simulink model "DRPLDM_2015a"  (R2015a)
settings: Solver=ode3  StartTime=0.0  StopTime=TimeVector(end)  FixedStep=Tsim  RelTol=1e-3
values from neighbouring files (symbols this model uses):
  EngUnits = 1    [RunModel.m]
  HILMode = 1    [RunModel.m]
  LeverMode = 1    [RunModel.m]
  Mode = 0    [RunModel.m]
  Mwm = 0.35    [RunModel.m]
  TCFaultSoftSim = 1    [RunModel.m]    (also in SetFaultSim.m)
  WhichCont = 2    [RunModel.m]
  WhichEngine = 1    [RunModel.m]
undefined symbols (not defined in the file or in its folder): FaultStartTime, FaultStopTime
libraries: Lib_Solve_ModelSource_TMATS x5, simulink x3
settings Model: Creator=antoniohadadeneto  LastModifiedBy=anton
settings DataIOCC: LimitDataPoints=off  SaveFormat=Dataset
settings HardwareCC: ProdBitPerPointer=64  ProdLargestAtomicFloat=Float  ProdIntDivRoundTo=Zero  ProdEndianess=LittleEndian  ProdHWDeviceType=Specified
settings GRTTargetCC: GeneratePreprocessorConditionals=Use local settings

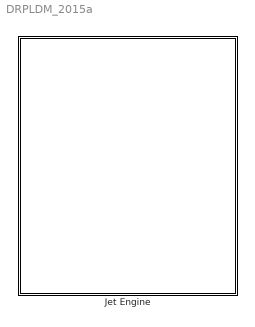
== system DRPLDM_2015a ==
  Jet Engine : Subsystem

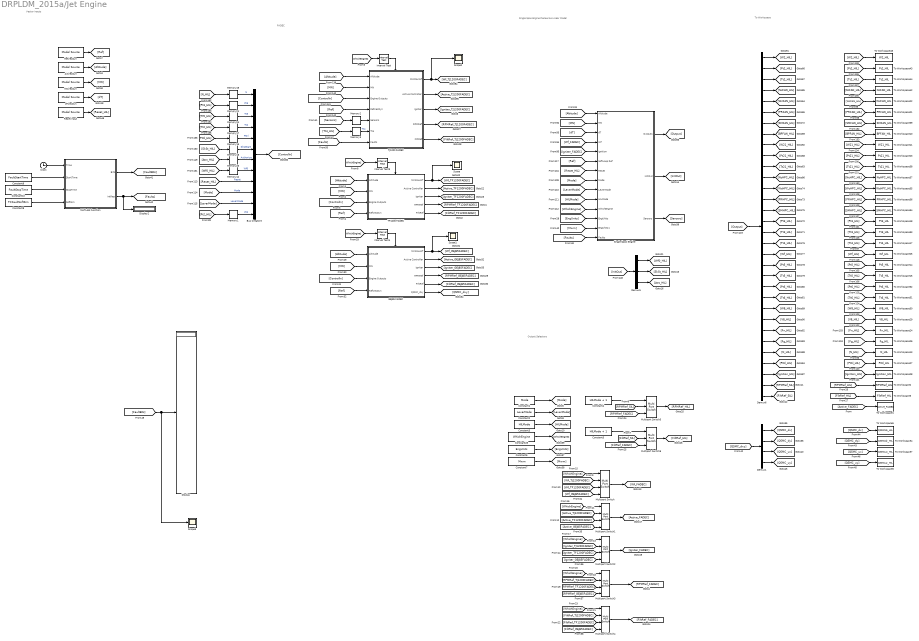
== system DRPLDM_2015a/Jet Engine ==
  note: Vector Inputs
  note: Single Spoo Engine
      | Piecewise
      | Linear Model
  note: To Workspace
  note: Output Selectors
  note: FADEC
  AltVecDyn : Lib_Solve_ModelSource_TMATS/Model Source  T_vec_M=TimeVector  input_array_M=AltVecDyn
  Bus Creator3 : BusCreator  Inputs=12
  Clock : Clock
  Constant1 : Constant  Value=Mode
  Constant10 : Constant  Value=FaultStopTime
  Constant2 : Constant  Value=LeverMode
  Constant25 : Constant  Value=WhichEngine
  Constant3 : Constant  Value=HILMode
  Constant4 : Constant  Value=HILMode + 1
  Constant5 : Constant  Value=HILMode + 1
  Constant6 : Constant  Value=EngUnits
  Constant7 : Constant  Value=Mwm
  Constant8 : Constant  Value=TCFaultSoftSim
  Constant9 : Constant  Value=FaultStartTime
  Demux1 : Demux
  Demux5 : Demux  Outputs=3
  Demux6 : Demux  Outputs=32
  Display : Display
  Display2 : Display
  GEJ85 FADEC : Subsystem  TreatAsAtomicUnit=on
  Interval Test : simulink/Logic and Bit Operations/Interval Test  IntervalClosedRight=on  uplimit=1.5  IntervalClosedLeft=on  lowlimit=0.5  OutDataTypeStr=boolean
  Interval Test3 : simulink/Logic and Bit Operations/Interval Test  IntervalClosedRight=on  uplimit=2.5  IntervalClosedLeft=on  lowlimit=1.5  OutDataTypeStr=boolean
  Interval Test4 : simulink/Logic and Bit Operations/Interval Test  IntervalClosedRight=on  uplimit=3.5  IntervalClosedLeft=on  lowlimit=2.5  OutDataTypeStr=boolean
  MATLAB Function : MATLAB Function  TreatAsAtomicUnit=on
      settings: PermitHierarchicalResolution=ParametersOnly
  MNVecDyn : Lib_Solve_ModelSource_TMATS/Model Source  T_vec_M=TimeVector  input_array_M=MNVecDyn
  Memory{1..3,12,15,17..19,21,24..25} (11 alike) : Memory
  Multiport Switch{,1..4} (5 alike) : MultiPortSwitch
  Multiport Switch5 : MultiPortSwitch  Inputs=2
  Multiport Switch6 : MultiPortSwitch  Inputs=2
  RefVecDyn : Lib_Solve_ModelSource_TMATS/Model Source  T_vec_M=TimeVector  input_array_M=RefVecDyn
  Reset Input : Lib_Solve_ModelSource_TMATS/Model Source  T_vec_M=TimeVector  input_array_M=ResetInput
  Scope{,1..3} (4 alike) : Scope
      Scope settings: TimeRange=auto  MaxDataPoints=5000  SaveToWorkspace=off  YMin=-1.00000  YMax=1.00000  SampleTime=-1
      Scope1 settings: TimeRange=auto  MaxDataPoints=5000  SaveToWorkspace=off  SaveName=ScopeData6  YMin=-0.03827  YMax=0.34443  SampleTime=-1
      Scope2 settings: TimeRange=auto  MaxDataPoints=5000  SaveToWorkspace=off  SaveName=ScopeData7  YMin=-1.00000  YMax=1.00000  SampleTime=-1
      Scope3 settings: TimeRange=auto  MaxDataPoints=5000  SaveToWorkspace=off  YMin=-0.125  YMax=1.125  SampleTime=-1
  Single Spool Engine : Subsystem  TreatAsAtomicUnit=on
  TF1200 FADEC : Subsystem  TreatAsAtomicUnit=on
  TJ1200 FADEC : Subsystem  TreatAsAtomicUnit=on
  To Workspace1 : ToWorkspace  VariableName=Active_FADEC  SampleTime=-1
  To Workspace13 : ToWorkspace  VariableName=N_HIL  SampleTime=-1
  To Workspace14 : ToWorkspace  VariableName=Pt5_HIL  SampleTime=-1
  To Workspace15 : ToWorkspace  VariableName=Tt5_HIL  SampleTime=-1
  To Workspace17 : ToWorkspace  VariableName=Tt4_HIL  SampleTime=-1
  To Workspace18 : ToWorkspace  VariableName=Pt3_HIL  SampleTime=-1
  To Workspace2 : ToWorkspace  VariableName=RPMRef_HIL  SampleTime=-1
  To Workspace21 : ToWorkspace  VariableName=PRFAN_HIL  SampleTime=-1
  To Workspace22 : ToWorkspace  VariableName=WcFAN_HIL  SampleTime=-1
  To Workspace23 : ToWorkspace  VariableName=Pt21_HIL  SampleTime=-1
  To Workspace24 : ToWorkspace  VariableName=Fn_HIL  SampleTime=-1
  To Workspace25 : ToWorkspace  VariableName=Wf_HIL  SampleTime=-1
  To Workspace26 : ToWorkspace  VariableName=Fg_HIL  SampleTime=-1
  To Workspace27 : ToWorkspace  VariableName=POil_HIL  SampleTime=-1
  To Workspace28 : ToWorkspace  VariableName=Ignition_HIL  SampleTime=-1
  To Workspace29 : ToWorkspace  VariableName=V8_HIL  SampleTime=-1
  To Workspace3 : ToWorkspace  VariableName=FiltRef_HIL  SampleTime=-1
  To Workspace30 : ToWorkspace  VariableName=W8_HIL  SampleTime=-1
  To Workspace31 : ToWorkspace  VariableName=Tt6_HIL  SampleTime=-1
  To Workspace32 : ToWorkspace  VariableName=Pt6_HIL  SampleTime=-1
  To Workspace33 : ToWorkspace  VariableName=Tt3_HIL  SampleTime=-1
  To Workspace34 : ToWorkspace  VariableName=SMHPC_HIL  SampleTime=-1
  To Workspace35 : ToWorkspace  VariableName=WcHPC_HIL  SampleTime=-1
  To Workspace36 : ToWorkspace  VariableName=PRHPC_HIL  SampleTime=-1
  To Workspace37 : ToWorkspace  VariableName=NcHPC_HIL  SampleTime=-1
  To Workspace38 : ToWorkspace  VariableName=Tt21_HIL  SampleTime=-1
  To Workspace39 : ToWorkspace  VariableName=SMFAN_HIL  SampleTime=-1
  To Workspace4 : ToWorkspace  VariableName=QSMCdy_HIL  SampleTime=-1
  To Workspace40 : ToWorkspace  VariableName=BPFAN_HIL  SampleTime=-1
  To Workspace41 : ToWorkspace  VariableName=W21_HIL  SampleTime=-1
  To Workspace42 : ToWorkspace  VariableName=NcFAN_HIL  SampleTime=-1
  To Workspace43 : ToWorkspace  VariableName=Pt2_HIL  SampleTime=-1
  To Workspace44 : ToWorkspace  VariableName=Tt2_HIL  SampleTime=-1
  To Workspace45 : ToWorkspace  VariableName=W2_HIL  SampleTime=-1
  To Workspace5 : ToWorkspace  VariableName=QSMCdx_HIL  SampleTime=-1
  To Workspace6 : ToWorkspace  VariableName=QSMCuy_HIL  SampleTime=-1
  To Workspace7 : ToWorkspace  VariableName=QSMCux_HIL  SampleTime=-1
  dTVecDyn : Lib_Solve_ModelSource_TMATS/Model Source  T_vec_M=TimeVector  input_array_M=dTVecDyn
  wires:
  [QSMC_uy] -> To Workspace6/1
  Demux6/29 -> [POil_HIL]
  [Pt5_HIL] -> To Workspace14/1
  Demux6/16 -> [Pt3_HIL]
  [Fn_HIL] -> To Workspace24/1
  [Reset_HIL] -> Single Spool Engine/7(Reset)
  Demux6/15 -> [SMHPC_HIL]
  [WhichEngine] -> Interval Test3/1
  [Wf_HIL] -> To Workspace25/1
  dTVecDyn/1 -> [dT]
  GEJ85 FADEC/2(Active Controller) -> [Active_GEJ85FADEC]
  [Pt3_HIL] -> To Workspace18/1
  Memory19/1 -> Bus Creator3/1  "N"
  [WcFAN_HIL] -> To Workspace22/1
  [NcHPC_HIL] -> To Workspace37/1
  [Tt3_HIL] -> To Workspace33/1
  [Active_FADEC] -> To Workspace1/1
  Interval Test3/1 -> TF1200 FADEC/Enable
  [W21_HIL] -> To Workspace41/1
  [WhichEngine] -> Interval Test/1
  Demux6/30 -> [Ignition_HIL]
  Interval Test/1 -> TJ1200 FADEC/Enable
  [Ignition_HIL] -> To Workspace28/1
  [Pt2_HIL] -> To Workspace43/1
  Constant2/1 -> [LeverMode]
  Memory1/1 -> Bus Creator3/12  "Pt2"
  [MN] -> TJ1200 FADEC/2(MN)
  [QSMC_dxy] -> Demux1/1
  TJ1200 FADEC/3(Igniter) -> [Igniter_TJ1200FADEC]
  [Tt21_HIL] -> To Workspace38/1
  GEJ85 FADEC/4(RPMRef) -> [RPMRef_GEJ85FADEC]
  Demux6/31 -> [RPMRef_SIL]
  Multiport Switch2/1 -> [Igniter_FADEC]
  Demux6/22 -> [Pt6_HIL]
  Constant3/1 -> [HILMode]
  Demux6/21 -> [Tt5_HIL]
  Demux6/17 -> [Tt3_HIL]
  [Pt6_HIL] -> To Workspace32/1
  Demux6/25 -> [V8_HIL]
  [Ref] -> Single Spool Engine/6(SoftLoop Ref)
  [Output] -> Demux6/1
  [N_HIL] -> To Workspace13/1
  Demux6/3 -> [Tt2_HIL]
  Demux6/32 -> [FiltRef_SIL]
  Demux6/23 -> [Tt6_HIL]
  Demux6/13 -> [WcHPC_HIL]
  Memory12/1 -> Bus Creator3/8  "Wf0"
  Multiport Switch/1 -> [Wf_FADEC]
  Memory21/1 -> Bus Creator3/2  "Pt3"
  TJ1200 FADEC/2(Active Controller) -> [Active_TJ1200FADEC]
  Demux6/24 -> [W8_HIL]
  Demux6/19 -> [Wf_HIL]
  [WhichEngine] -> Multiport Switch2/1
  [SMHPC_HIL] -> To Workspace34/1
  [Igniter_TJ1200FADEC] -> Multiport Switch2/2
  Demux6/26 -> [Fn_HIL]
  [Altitude] -> GEJ85 FADEC/1(Altitude)
  [ControlIn] -> TJ1200 FADEC/3(Engine Outputs)
  [Tt6_HIL] -> To Workspace31/1
  [PRHPC_HIL] -> To Workspace36/1
  [NcFAN_HIL] -> To Workspace42/1
  [W2_HIL] -> To Workspace45/1
  [ControlIn] -> TF1200 FADEC/3(Engine Outputs)
  [Tt2_HIL] -> To Workspace44/1
  Interval Test4/1 -> GEJ85 FADEC/Enable
  [FiltRef_TJ1200FADEC] -> Multiport Switch4/2
  [RPMRef_TF1200FADEC] -> Multiport Switch3/3
  Demux5/1 -> [Wf0_HIL]
  [Pt3_HIL] -> Memory21/1
  [Ref] -> TJ1200 FADEC/4(RefVecDyn)
  [ControlIn] -> GEJ85 FADEC/3(Engine Outputs)
  TJ1200 FADEC/1(MinMaxWf) -> Scope2/1, [Wf_TJ1200FADEC]
  [Altitude] -> TJ1200 FADEC/1(Altitude)
  Constant25/1 -> [WhichEngine]
  [LeverMode] -> Bus Creator3/11  "LeverMode"
  Memory25/1 -> Bus Creator3/7  "Authorize"
  [Mode] -> Bus Creator3/10  "Mode"
  [Reset_HIL] -> Bus Creator3/9  "Reset"
  [W8_HIL] -> To Workspace30/1
  [V8_HIL] -> To Workspace29/1
  TF1200 FADEC/1(MinMaxWf) -> Scope/1, [Wf_TF1200FADEC]
  [SMFAN_HIL] -> To Workspace39/1
  Memory15/1 -> Bus Creator3/5  "POil"
  Demux6/28 -> [N_HIL]
  [Wf0_HIL] -> Memory12/1
  TF1200 FADEC/2(Active Controller) -> [Active_TF1200FADEC]
  Demux5/2 -> [SkSt_HIL]
  Demux6/6 -> [PRFAN_HIL]
  [Ref] -> TF1200 FADEC/4(RefVecDyn)
  Memory17/1 -> Bus Creator3/4  "Tt2"
  TF1200 FADEC/3(Igniter) -> [Igniter_TF1200FADEC]
  [N_HIL] -> Memory19/1
  [MN] -> GEJ85 FADEC/2(MN)
  [MN] -> TF1200 FADEC/2(MN)
  Demux6/10 -> [Pt21_HIL]
  GEJ85 FADEC/3(Igniter) -> [Igniter_GEJ85FADEC]
  Demux6/11 -> [Tt21_HIL]
  MNVecDyn/1 -> [MN]
  AltVecDyn/1 -> [Altitude]
  Demux6/12 -> [NcHPC_HIL]
  [RPMRef_TJ1200FADEC] -> Multiport Switch3/2
  [Altitude] -> TF1200 FADEC/1(Altitude)
  Single Spool Engine/1(Outputs) -> [Output]
  [dT] -> Single Spool Engine/3(dT)
  Constant5/1 -> Multiport Switch6/1
  [Tt5_HIL] -> To Workspace15/1
  [Pt21_HIL] -> To Workspace23/1
  [Tt4_HIL] -> To Workspace17/1
  [PRFAN_HIL] -> To Workspace21/1
  [Wf_FADEC] -> Single Spool Engine/4(Wf)
  [Altitude] -> Single Spool Engine/1(Altitude)
  Demux6/1 -> [W2_HIL]
  Demux6/5 -> [WcFAN_HIL]
  [Fg_HIL] -> To Workspace26/1
  Demux6/9 -> [W21_HIL]
  [Mode] -> Single Spool Engine/8(Mode)
  Demux1/3 -> [QSMC_ux]
  [FiltRef_GEJ85FADEC] -> Multiport Switch4/4
  [WhichEngine] -> Interval Test4/1
  [Wf_TF1200FADEC] -> Multiport Switch/3
  TF1200 FADEC/5(FiltRef) -> [FiltRef_TF1200FADEC]
  Constant4/1 -> Multiport Switch5/1
  [WhichEngine] -> Multiport Switch4/1
  [Wf_TJ1200FADEC] -> Multiport Switch/2
  Reset Input/1 -> [Reset_HIL]
  [WhichEngine] -> Multiport Switch3/1
  [WhichEngine] -> Multiport Switch1/1
  [Active_TF1200FADEC] -> Multiport Switch1/3
  [Active_GEJ85FADEC] -> Multiport Switch1/4
  [WhichEngine] -> Multiport Switch/1
  [SkSt_HIL] -> Memory18/1
  [MN] -> Single Spool Engine/2(MN)
  [FiltRef_SIL] -> Multiport Switch6/2
  Memory24/1 -> Bus Creator3/3  "Tt5"
  [RPMRef_SIL] -> Multiport Switch5/2
  Demux5/3 -> [Atrz_HIL]
  [Igniter_FADEC] -> Single Spool Engine/5(Ignition)
  [FiltRef_HIL] -> To Workspace3/1
  [RPMRef_FADEC] -> Multiport Switch5/3
  [WhichEngine] -> Single Spool Engine/11(WhichEngine)
  [Active_TJ1200FADEC] -> Multiport Switch1/2
  [FiltRef_TF1200FADEC] -> Multiport Switch4/3
  [FiltRef_FADEC] -> Multiport Switch6/3
  GEJ85 FADEC/5(FiltRef) -> [FiltRef_GEJ85FADEC]
  TJ1200 FADEC/4(RPMRef) -> [RPMRef_TJ1200FADEC]
  [Igniter_TF1200FADEC] -> Multiport Switch2/3
  TF1200 FADEC/4(RPMRef) -> [RPMRef_TF1200FADEC]
  [POil_HIL] -> To Workspace27/1
  Demux6/7 -> [SMFAN_HIL]
  Demux6/20 -> [Pt5_HIL]
  [WcHPC_HIL] -> To Workspace35/1
  [Ref] -> GEJ85 FADEC/4(RefVecDyn)
  GEJ85 FADEC/1(MinMaxWf) -> Scope1/1, [Wf_GEJ85FADEC]
  Multiport Switch6/1 -> [FiltRef_HIL]
  Multiport Switch3/1 -> [RPMRef_FADEC]
  [Tt5_HIL] -> Memory24/1
  Multiport Switch5/1 -> [RPMRef_HIL]
  [Wf_GEJ85FADEC] -> Multiport Switch/4
  [BPFAN_HIL] -> To Workspace40/1
  Demux6/8 -> [BPFAN_HIL]
  [Atrz_HIL] -> Memory25/1
  Demux6/27 -> [Fg_HIL]
  [Igniter_GEJ85FADEC] -> Multiport Switch2/4
  [RPMRef_GEJ85FADEC] -> Multiport Switch3/4
  [Tt2_HIL] -> Memory17/1
  [QSMC_dy] -> To Workspace4/1
  RefVecDyn/1 -> [Ref]
  Demux1/2 -> [QSMC_dy]
  Demux6/18 -> [Tt4_HIL]
  Demux6/4 -> [NcFAN_HIL]
  Multiport Switch1/1 -> [Active_FADEC]
  Constant1/1 -> [Mode]
  [QSMC_dx] -> To Workspace5/1
  Single Spool Engine/2(InitOut) -> [InitOut]
  Demux6/2 -> [Pt2_HIL]
  [QSMC_ux] -> To Workspace7/1
  GEJ85 FADEC/6(QSMC_dxy) -> [QSMC_dxy]
  Demux1/1 -> [QSMC_dx]
  [InitOut] -> Demux5/1
  Demux1/4 -> [QSMC_uy]
  TJ1200 FADEC/5(FiltRef) -> [FiltRef_TJ1200FADEC]
  Bus Creator3/1 -> [ControlIn]
  Multiport Switch4/1 -> [FiltRef_FADEC]
  [LeverMode] -> Single Spool Engine/9(LeverMode)
  [Pt2_HIL] -> Memory1/1
  Memory18/1 -> Bus Creator3/6  "SkipStart"
  [POil_HIL] -> Memory15/1
  [RPMRef_HIL] -> To Workspace2/1
  Demux6/14 -> [PRHPC_HIL]
  [HILMode] -> Single Spool Engine/10(HILMode)
  Constant6/1 -> [EngUnits]
  [EngUnits] -> Single Spool Engine/12(EngUhits)
  [Mwm] -> Single Spool Engine/13(EngUhits1)
  Constant7/1 -> [Mwm]
  Single Spool Engine/3(Sensors) -> [Sensors]
  [Sensors] -> Memory2/1
  Memory2/1 -> TJ1200 FADEC/5(Sensors)
  Memory3/1 -> TJ1200 FADEC/6(Tt4)  "Tt4"
  [Tt4_HIL] -> Memory3/1
  [Faults] -> Single Spool Engine/14(Faults)
  [FaultBits] -> Scope3/1, Display/1
  Clock/1 -> MATLAB Function/1(Time)
  Constant9/1 -> MATLAB Function/2(StartTime)
  Constant10/1 -> MATLAB Function/3(StopTime)
  MATLAB Function/1(Bits) -> [FaultBits]
  MATLAB Function/2(IntRep) -> [Faults], Display2/1
  [Faults] -> TJ1200 FADEC/7(Faults)
  Constant8/1 -> MATLAB Function/4(SoftSim)

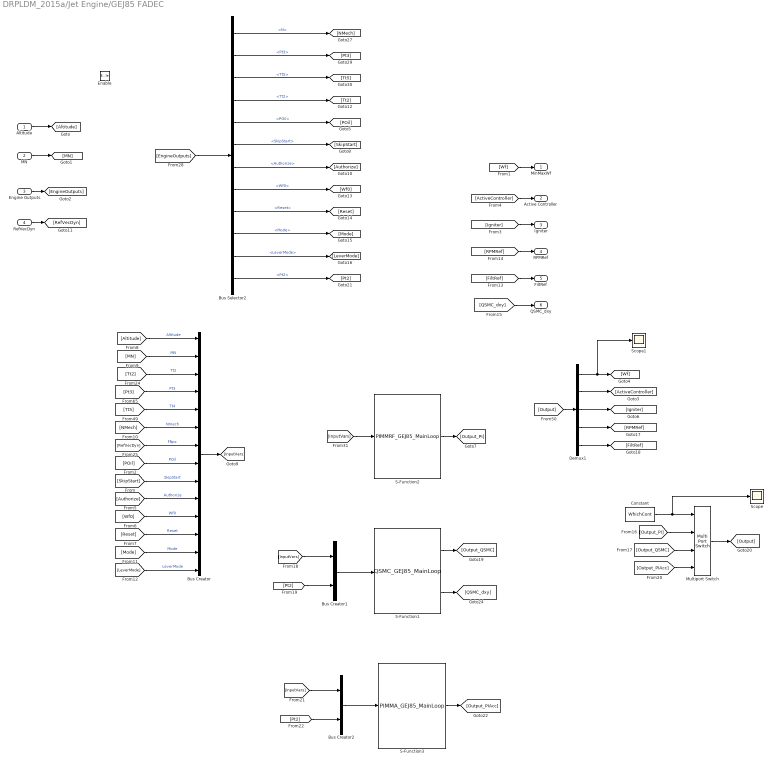
== system DRPLDM_2015a/Jet Engine/GEJ85 FADEC ==
  Altitude : Inport
  MN : Inport  Port=2
  Engine Outputs : Inport  Port=3
  RefVecDyn : Inport  Port=4
  Enable : EnablePort
  Bus Creator : BusCreator  Inputs=14
  Bus Creator1 : BusCreator  Inputs=2
  Bus Creator2 : BusCreator  Inputs=2
  Bus Selector2 : BusSelector  OutputSignals=N,Pt3,Tt5,Tt2,POil,SkipStart,Authorize,Wf0,Reset,Mode,LeverMode,Pt2
  Constant : Constant  Value=WhichCont
  Demux1 : Demux  Outputs=5
  Multiport Switch : MultiPortSwitch
  S-Function1 : S-Function  FunctionName=QSMC_GEJ85_MainLoop  SFunctionDeploymentMode=off  EnableBusSupport=off
  S-Function2 : S-Function  FunctionName=PIMMRF_GEJ85_MainLoop  SFunctionDeploymentMode=off  EnableBusSupport=off
  S-Function3 : S-Function  FunctionName=PIMMA_GEJ85_MainLoop  SFunctionDeploymentMode=off  EnableBusSupport=off
  Scope : Scope
      settings: TimeRange=auto  MaxDataPoints=5000  SaveToWorkspace=off  YMin=1.00000  YMax=3.00000  SampleTime=-1
  Scope1 : Scope
      settings: TimeRange=auto  MaxDataPoints=5000  SaveToWorkspace=off  SaveName=ScopeData2  YMin=-0.03465  YMax=0.31188  SampleTime=-1
  MinMaxWf : Outport
  Active Controller : Outport  Port=2  InitialOutput=0
  Igniter : Outport  Port=3  InitialOutput=0
  RPMRef : Outport  Port=4  InitialOutput=0
  FiltRef : Outport  Port=5  InitialOutput=0
  QSMC_dxy : Outport  Port=6  InitialOutput=0
  wires:
  Demux1/5 -> [FiltRef]
  Demux1/4 -> [RPMRef]
  [FiltRef] -> FiltRef/1
  [RPMRef] -> RPMRef/1
  Bus Selector2/4 -> [Tt2]  "<Tt2>"
  Altitude/1 -> [Altitude]
  MN/1 -> [MN]
  Engine Outputs/1 -> [EngineOutputs]
  RefVecDyn/1 -> [RefVecDyn]
  [EngineOutputs] -> Bus Selector2/1
  Bus Selector2/1 -> [NMech]  "<N>"
  Bus Selector2/2 -> [Pt3]  "<Pt3>"
  Bus Selector2/3 -> [Tt5]  "<Tt5>"
  [Wf] -> MinMaxWf/1
  [ActiveController] -> Active Controller/1
  [Altitude] -> Bus Creator/1  "Altitude"
  [MN] -> Bus Creator/2  "MN"
  Bus Creator/1 -> [InputVars]
  [InputVars] -> S-Function2/1
  S-Function2/1 -> [Output_PI]
  [Output] -> Demux1/1
  Demux1/1 -> Scope1/1, [Wf]
  Demux1/2 -> [ActiveController]
  [Tt2] -> Bus Creator/3  "Tt2"
  [Pt3] -> Bus Creator/4  "Pt3"
  [Tt5] -> Bus Creator/5  "Tt4"
  [NMech] -> Bus Creator/6  "Nmech"
  [RefVecDyn] -> Bus Creator/7  "FNpc"
  Bus Selector2/5 -> [POil]  "<POil>"
  [POil] -> Bus Creator/8  "POil"
  Demux1/3 -> [Igniter]
  [Igniter] -> Igniter/1
  Bus Selector2/6 -> [SkipStart]  "<SkipStart>"
  [SkipStart] -> Bus Creator/9  "SkipStart"
  Bus Selector2/7 -> [Authorize]  "<Authorize>"
  Bus Selector2/8 -> [Wf0]  "<Wf0>"
  [Authorize] -> Bus Creator/10  "Authorize"
  [Wf0] -> Bus Creator/11  "Wf0"
  Bus Selector2/9 -> [Reset]  "<Reset>"
  [Reset] -> Bus Creator/12  "Reset"
  Bus Selector2/10 -> [Mode]  "<Mode>"
  Bus Selector2/11 -> [LeverMode]  "<LeverMode>"
  [Mode] -> Bus Creator/13  "Mode"
  [LeverMode] -> Bus Creator/14  "LeverMode"
  Bus Creator1/1 -> S-Function1/1
  S-Function1/1 -> [Output_QSMC]
  [Output_QSMC] -> Multiport Switch/3
  [Output_PI] -> Multiport Switch/2
  Constant/1 -> Scope/1, Multiport Switch/1
  Multiport Switch/1 -> [Output]
  [InputVars] -> Bus Creator1/1
  Bus Selector2/12 -> [Pt2]  "<Pt2>"
  [Pt2] -> Bus Creator1/2
  S-Function1/2 -> [QSMC_dxy]
  [QSMC_dxy] -> QSMC_dxy/1
  S-Function3/1 -> [Output_PIAcc]
  [Pt2] -> Bus Creator2/2
  [InputVars] -> Bus Creator2/1
  Bus Creator2/1 -> S-Function3/1
  [Output_PIAcc] -> Multiport Switch/4

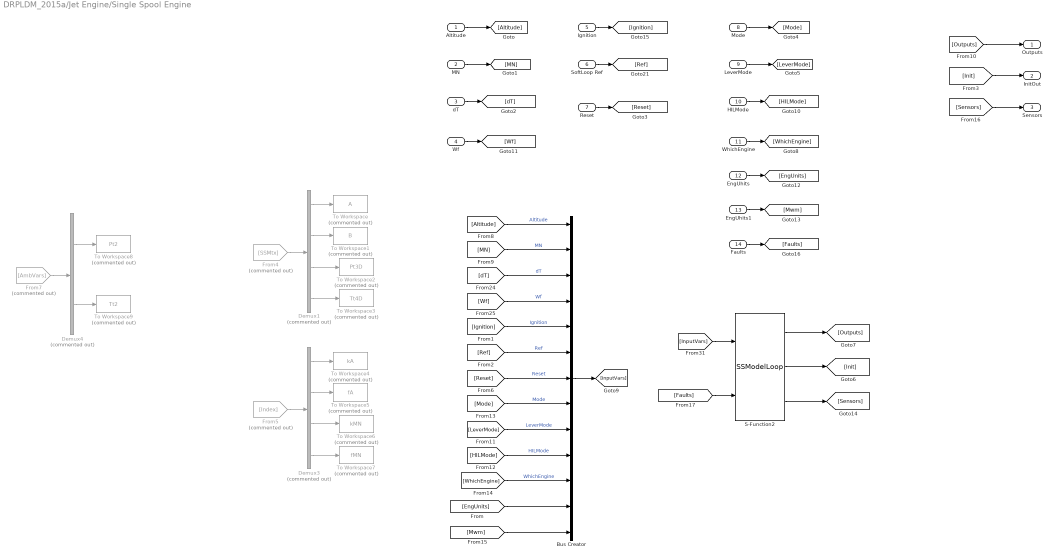
== system DRPLDM_2015a/Jet Engine/Single Spool Engine ==
  Altitude : Inport
  MN : Inport  Port=2
  dT : Inport  Port=3
  Wf : Inport  Port=4
  Ignition : Inport  Port=5
  SoftLoop Ref : Inport  Port=6
  Reset : Inport  Port=7
  Mode : Inport  Port=8
  LeverMode : Inport  Port=9
  HILMode : Inport  Port=10
  WhichEngine : Inport  Port=11
  EngUhits : Inport  Port=12
  EngUhits1 : Inport  Port=13
  Faults : Inport  Port=14
  Bus Creator : BusCreator  Inputs=13
  Demux1 : Demux  Commented=on
  Demux3 : Demux  Commented=on
  Demux4 : Demux  Commented=on  Outputs=2
  From4 : From  Commented=on  GotoTag=SSMtx
  From5 : From  Commented=on  GotoTag=Index
  From7 : From  Commented=on  GotoTag=AmbVars
  S-Function2 : S-Function  FunctionName=SSModelLoop  SFunctionDeploymentMode=off  EnableBusSupport=off
  To Workspace : ToWorkspace  Commented=on  VariableName=A  SampleTime=-1
  To Workspace1 : ToWorkspace  Commented=on  VariableName=B  SampleTime=-1
  To Workspace2 : ToWorkspace  Commented=on  VariableName=Pt3D  SampleTime=-1
  To Workspace3 : ToWorkspace  Commented=on  VariableName=Tt4D  SampleTime=-1
  To Workspace4 : ToWorkspace  Commented=on  VariableName=kA  SampleTime=-1
  To Workspace5 : ToWorkspace  Commented=on  VariableName=fA  SampleTime=-1
  To Workspace6 : ToWorkspace  Commented=on  VariableName=kMN  SampleTime=-1
  To Workspace7 : ToWorkspace  Commented=on  VariableName=fMN  SampleTime=-1
  To Workspace8 : ToWorkspace  Commented=on  VariableName=Pt2  SampleTime=-1
  To Workspace9 : ToWorkspace  Commented=on  VariableName=Tt2  SampleTime=-1
  Outputs : Outport
  InitOut : Outport  Port=2
  Sensors : Outport  Port=3
  wires:
  Ignition/1 -> [Ignition]
  [Outputs] -> Outputs/1
  Demux4/1 -> To Workspace8/1
  Demux4/2 -> To Workspace9/1
  From7/1 -> Demux4/1
  From5/1 -> Demux3/1
  Demux3/3 -> To Workspace6/1
  Demux3/4 -> To Workspace7/1
  Demux3/2 -> To Workspace5/1
  Demux3/1 -> To Workspace4/1
  From4/1 -> Demux1/1
  Demux1/3 -> To Workspace2/1
  Demux1/4 -> To Workspace3/1
  Demux1/2 -> To Workspace1/1
  Demux1/1 -> To Workspace/1
  Altitude/1 -> [Altitude]
  MN/1 -> [MN]
  dT/1 -> [dT]
  Wf/1 -> [Wf]
  [Altitude] -> Bus Creator/1  "Altitude"
  [MN] -> Bus Creator/2  "MN"
  Bus Creator/1 -> [InputVars]
  [dT] -> Bus Creator/3  "dT"
  [Wf] -> Bus Creator/4  "Wf"
  [Ignition] -> Bus Creator/5  "Ignition"
  [InputVars] -> S-Function2/1
  S-Function2/1 -> [Outputs]
  SoftLoop Ref/1 -> [Ref]
  [Ref] -> Bus Creator/6  "Ref"
  S-Function2/2 -> [Init]
  [Init] -> InitOut/1
  [Reset] -> Bus Creator/7  "Reset"
  Reset/1 -> [Reset]
  WhichEngine/1 -> [WhichEngine]
  HILMode/1 -> [HILMode]
  LeverMode/1 -> [LeverMode]
  Mode/1 -> [Mode]
  [Mode] -> Bus Creator/8  "Mode"
  [LeverMode] -> Bus Creator/9  "LeverMode"
  [HILMode] -> Bus Creator/10  "HILMode"
  [WhichEngine] -> Bus Creator/11  "WhichEngine"
  EngUhits/1 -> [EngUnits]
  [EngUnits] -> Bus Creator/12
  [Mwm] -> Bus Creator/13
  EngUhits1/1 -> [Mwm]
  S-Function2/3 -> [Sensors]
  [Sensors] -> Sensors/1
  Faults/1 -> [Faults]
  [Faults] -> S-Function2/2

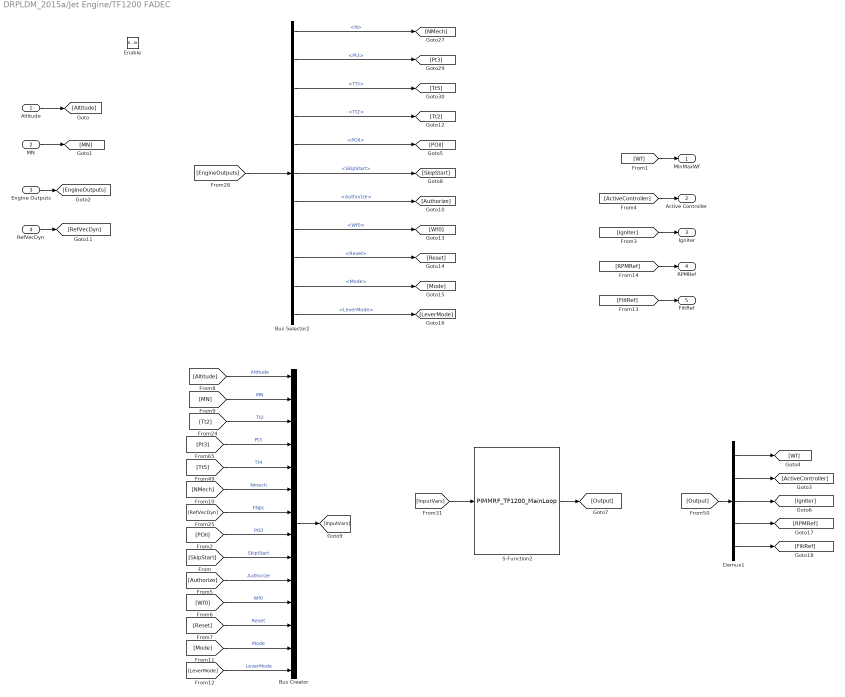
== system DRPLDM_2015a/Jet Engine/TF1200 FADEC ==
  Altitude : Inport
  MN : Inport  Port=2
  Engine Outputs : Inport  Port=3
  RefVecDyn : Inport  Port=4
  Enable : EnablePort
  Bus Creator : BusCreator  Inputs=14
  Bus Selector2 : BusSelector  OutputSignals=N,Pt3,Tt5,Tt2,POil,SkipStart,Authorize,Wf0,Reset,Mode,LeverMode
  Demux1 : Demux  Outputs=5
  S-Function2 : S-Function  FunctionName=PIMMRF_TF1200_MainLoop  SFunctionDeploymentMode=off  EnableBusSupport=off
  MinMaxWf : Outport
  Active Controller : Outport  Port=2  InitialOutput=0
  Igniter : Outport  Port=3  InitialOutput=0
  RPMRef : Outport  Port=4  InitialOutput=0
  FiltRef : Outport  Port=5  InitialOutput=0
  wires:
  [LeverMode] -> Bus Creator/14  "LeverMode"
  [Mode] -> Bus Creator/13  "Mode"
  Bus Selector2/11 -> [LeverMode]  "<LeverMode>"
  Bus Selector2/10 -> [Mode]  "<Mode>"
  [Reset] -> Bus Creator/12  "Reset"
  Bus Selector2/9 -> [Reset]  "<Reset>"
  [Wf0] -> Bus Creator/11  "Wf0"
  [Authorize] -> Bus Creator/10  "Authorize"
  Bus Selector2/8 -> [Wf0]  "<Wf0>"
  Bus Selector2/7 -> [Authorize]  "<Authorize>"
  [SkipStart] -> Bus Creator/9  "SkipStart"
  Bus Selector2/6 -> [SkipStart]  "<SkipStart>"
  [Igniter] -> Igniter/1
  Demux1/3 -> [Igniter]
  [POil] -> Bus Creator/8  "POil"
  Bus Selector2/5 -> [POil]  "<POil>"
  [RefVecDyn] -> Bus Creator/7  "FNpc"
  [NMech] -> Bus Creator/6  "Nmech"
  [Tt5] -> Bus Creator/5  "Tt4"
  [Pt3] -> Bus Creator/4  "Pt3"
  [Tt2] -> Bus Creator/3  "Tt2"
  Demux1/2 -> [ActiveController]
  Demux1/1 -> [Wf]
  [Output] -> Demux1/1
  S-Function2/1 -> [Output]
  [InputVars] -> S-Function2/1
  Bus Creator/1 -> [InputVars]
  [MN] -> Bus Creator/2  "MN"
  [Altitude] -> Bus Creator/1  "Altitude"
  [ActiveController] -> Active Controller/1
  [Wf] -> MinMaxWf/1
  Bus Selector2/3 -> [Tt5]  "<Tt5>"
  Bus Selector2/2 -> [Pt3]  "<Pt3>"
  Bus Selector2/1 -> [NMech]  "<N>"
  [EngineOutputs] -> Bus Selector2/1
  RefVecDyn/1 -> [RefVecDyn]
  Engine Outputs/1 -> [EngineOutputs]
  MN/1 -> [MN]
  Altitude/1 -> [Altitude]
  Bus Selector2/4 -> [Tt2]  "<Tt2>"
  [RPMRef] -> RPMRef/1
  [FiltRef] -> FiltRef/1
  Demux1/4 -> [RPMRef]
  Demux1/5 -> [FiltRef]

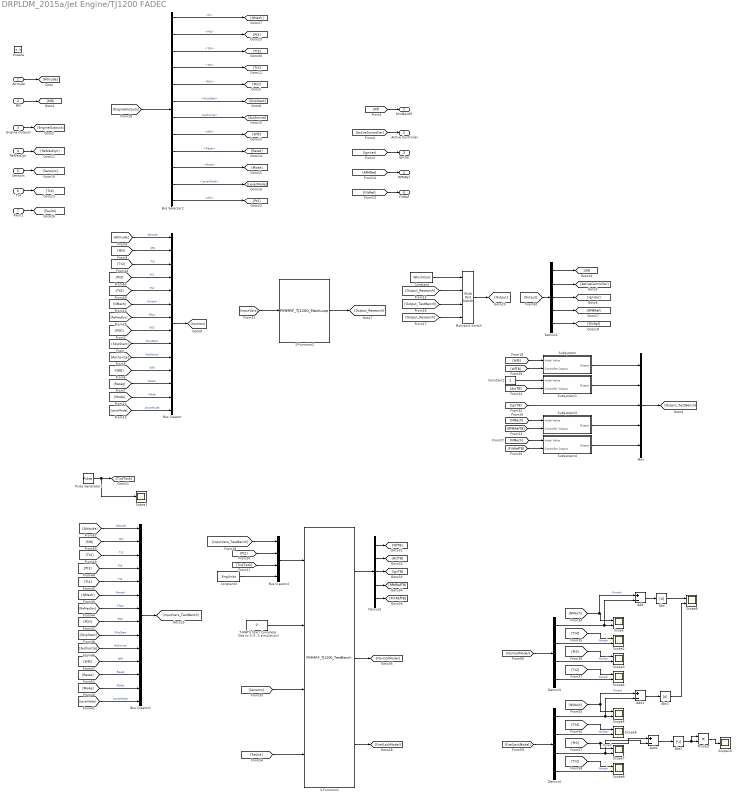
== system DRPLDM_2015a/Jet Engine/TJ1200 FADEC ==
  Altitude : Inport
  MN : Inport  Port=2
  Engine Outputs : Inport  Port=3
  RefVecDyn : Inport  Port=4
  Sensors : Inport  Port=5
  Tt4 : Inport  Port=6
  Faults : Inport  Port=7
  Enable : EnablePort
  Abs : Abs
  Abs1 : Abs
  Abs2 : Abs
  Add : Sum  Inputs=+-
  Add1 : Sum  Inputs=+-
  Add2 : Sum  Inputs=+-
  Bus Creator : BusCreator  Inputs=14
  Bus Creator1 : BusCreator  Inputs=14
  Bus Creator2 : BusCreator  Inputs=4
  Bus Selector2 : BusSelector  OutputSignals=N,Pt3,Tt5,Tt2,POil,SkipStart,Authorize,Wf0,Reset,Mode,LeverMode,Pt2
  Constant : Constant  Value=WhichCont
  Constant2 : Constant
  Constant3 : Constant  Value=EngUnits
  Demux1 : Demux  Outputs=5
  Demux2 : Demux  Outputs=5
  Demux3 : Demux
  Demux4 : Demux
  Multiport Switch : MultiPortSwitch
  Mux : Mux  Inputs=5
  Product : Product
  Pulse Generator1 : DiscretePulseGenerator  PulseType=Time based  Period=2 * 0.001 * 200  PulseWidth=50
  S-Function1 : S-Function  FunctionName=PIMMRF_TJ1200_TestBench  SFunctionDeploymentMode=off  EnableBusSupport=off
  S-Function2 : S-Function  FunctionName=PIMMRF_TJ1200_MainLoop  SFunctionDeploymentMode=off  EnableBusSupport=off
  Scope{,2..9} (9 alike) : Scope  NumInputPorts=2
      Scope settings: TimeRange=auto  MaxDataPoints=5000  SaveToWorkspace=off  YMin=-4359.66321~-5  YMax=27489.0227~5  SampleTime=-1
      Scope2 settings: TimeRange=auto  MaxDataPoints=5000  SaveToWorkspace=off  SaveName=ScopeData2  YMin=-175.79542~-5  YMax=1582.1588~5  SampleTime=-1
      Scope3 settings: TimeRange=auto  MaxDataPoints=5000  SaveToWorkspace=off  SaveName=ScopeData3  YMin=-67762.95694~-5  YMax=609866.61249~5  SampleTime=-1
      Scope4 settings: TimeRange=auto  MaxDataPoints=5000  SaveToWorkspace=off  SaveName=ScopeData4  YMin=-41.51665~-5  YMax=373.64989~5  SampleTime=-1
      Scope5 settings: TimeRange=auto  MaxDataPoints=5000  SaveToWorkspace=off  YMin=-4359.66321~-5  YMax=27489.0227~5  SampleTime=-1
      Scope6 settings: TimeRange=auto  MaxDataPoints=5000  SaveToWorkspace=off  SaveName=ScopeData2  YMin=84.38547~-5  YMax=1308.61996~5  SampleTime=-1
      Scope7 settings: TimeRange=auto  MaxDataPoints=5000  SaveToWorkspace=off  SaveName=ScopeData3  YMin=129347.02545~-5  YMax=453881.88091~5  SampleTime=-1
      Scope8 settings: TimeRange=auto  MaxDataPoints=5000  SaveToWorkspace=off  SaveName=ScopeData4  YMin=-41.51665~-5  YMax=373.64989~5  SampleTime=-1
      Scope9 settings: TimeRange=auto  MaxDataPoints=5000  SaveToWorkspace=off  YMin=-262.24287~-5  YMax=3401.91833~5  SampleTime=-1
  Scope1 : Scope
      settings: TimeRange=auto  MaxDataPoints=5000  SaveToWorkspace=off  YMin=-0.04804  YMax=1.04517  SampleTime=-1
  Scope10 : Scope
      settings: TimeRange=auto  MaxDataPoints=5000  SaveToWorkspace=off  YMin=84.38547  YMax=1308.61996  SampleTime=-1
  Subsystem : Subsystem
  Subsystem1 : Subsystem
  Subsystem3 : Subsystem
  Subsystem4 : Subsystem
  T-MATS Start Complete (Set to 0 if not T-MATS simulation) : Constant  Value=0
  MinMaxWf : Outport
  Active Controller : Outport  Port=2  InitialOutput=0
  Igniter : Outport  Port=3  InitialOutput=0
  RPMRef : Outport  Port=4  InitialOutput=0
  FiltRef : Outport  Port=5  InitialOutput=0
  wires:
  Bus Selector2/4 -> [Tt2]  "<Tt2>"
  Altitude/1 -> [Altitude]
  MN/1 -> [MN]
  Engine Outputs/1 -> [EngineOutputs]
  RefVecDyn/1 -> [RefVecDyn]
  [EngineOutputs] -> Bus Selector2/1
  Bus Selector2/1 -> [NMech]  "<N>"
  Bus Selector2/2 -> [Pt3]  "<Pt3>"
  Bus Selector2/3 -> [Tt5]  "<Tt5>"
  [Wf] -> MinMaxWf/1
  [ActiveController] -> Active Controller/1
  [Altitude] -> Bus Creator/1  "Altitude"
  [MN] -> Bus Creator/2  "MN"
  Bus Creator/1 -> [InputVars]
  [InputVars] -> S-Function2/1
  S-Function2/1 -> [Output_Research]
  [Output] -> Demux1/1
  Demux1/2 -> [ActiveController]
  [Tt2] -> Bus Creator/3  "Tt2"
  [Pt3] -> Bus Creator/4  "Pt3"
  [Tt5] -> Bus Creator/5  "Tt4"
  [NMech] -> Bus Creator/6  "Nmech"
  [RefVecDyn] -> Bus Creator/7  "FNpc"
  Bus Selector2/5 -> [POil]  "<POil>"
  [POil] -> Bus Creator/8  "POil"
  Demux1/3 -> [Igniter]
  [Igniter] -> Igniter/1
  Bus Selector2/6 -> [SkipStart]  "<SkipStart>"
  [SkipStart] -> Bus Creator/9  "SkipStart"
  Bus Selector2/7 -> [Authorize]  "<Authorize>"
  Bus Selector2/8 -> [Wf0]  "<Wf0>"
  [Authorize] -> Bus Creator/10  "Authorize"
  [Wf0] -> Bus Creator/11  "Wf0"
  Bus Selector2/9 -> [Reset]  "<Reset>"
  [Reset] -> Bus Creator/12  "Reset"
  Bus Selector2/10 -> [Mode]  "<Mode>"
  Bus Selector2/11 -> [LeverMode]  "<LeverMode>"
  [Mode] -> Bus Creator/13  "Mode"
  [LeverMode] -> Bus Creator/14  "LeverMode"
  Demux1/4 -> [RPMRef]
  Demux1/5 -> [FiltRef]
  [FiltRef] -> FiltRef/1
  [RPMRef] -> RPMRef/1
  [Output_TestBench] -> Multiport Switch/3
  Multiport Switch/1 -> [Output]
  [Output_Research] -> Multiport Switch/4
  [Output_Research] -> Multiport Switch/2
  Constant/1 -> Multiport Switch/1
  Pulse Generator1/1 -> Scope1/1, [TickTack]
  [InputVars_TestBench] -> Bus Creator2/1
  Bus Creator2/1 -> S-Function1/1
  [TickTack] -> Bus Creator2/3
  [Pt2] -> Bus Creator2/2
  Bus Selector2/12 -> [Pt2]  "<Pt2>"
  T-MATS Start Complete (Set to 0 if not T-MATS simulation)/1 -> S-Function1/2
  S-Function1/1 -> Demux2/1
  Demux1/1 -> [Wf]
  Subsystem/1(Output) -> Mux/1
  [Wf0] -> Subsystem/1(Initial Value)
  Constant2/1 -> Subsystem1/1(Initial Value)
  Subsystem1/1(Output) -> Mux/2
  [NMech] -> Subsystem3/1(Initial Value)
  Subsystem3/1(Output) -> Mux/4
  Subsystem4/1(Output) -> Mux/5
  [NMech] -> Subsystem4/1(Initial Value)
  [WfTB] -> Subsystem/2(Controller Output)
  Demux2/1 -> [WfTB]
  Demux2/2 -> [ActTB]
  Demux2/3 -> [IgnTB]
  Demux2/4 -> [RPMRefTB]
  Demux2/5 -> [FiltRefTB]
  [ActTB] -> Subsystem1/2(Controller Output)
  [RPMRefTB] -> Subsystem3/2(Controller Output)
  [FiltRefTB] -> Subsystem4/2(Controller Output)
  Mux/1 -> [Output_TestBench]
  [IgnTB] -> Mux/3
  Constant3/1 -> Bus Creator2/4
  Sensors/1 -> [Sensors]
  [Sensors] -> S-Function1/3
  S-Function1/2 -> [NormalModel]
  [NMech] -> Add/1, Scope/1  "Nmech"
  Demux3/1 -> Add/2, Scope/2
  Demux3/2 -> Scope2/2
  Demux3/3 -> Scope3/2
  Demux3/4 -> Scope4/2
  [Tt4] -> Scope2/1  "Nmech"
  [Pt3] -> Scope3/1  "Nmech"
  [Tt2] -> Scope4/1  "Nmech"
  Tt4/1 -> [Tt4]
  [LeverMode] -> Bus Creator1/14  "LeverMode"
  [Mode] -> Bus Creator1/13  "Mode"
  [Reset] -> Bus Creator1/12  "Reset"
  [Wf0] -> Bus Creator1/11  "Wf0"
  [Authorize] -> Bus Creator1/10  "Authorize"
  [SkipStart] -> Bus Creator1/9  "SkipStart"
  [POil] -> Bus Creator1/8  "POil"
  [RefVecDyn] -> Bus Creator1/7  "FNpc"
  [NMech] -> Bus Creator1/6  "Nmech"
  [Tt4] -> Bus Creator1/5  "Tt4"
  [Pt3] -> Bus Creator1/4  "Pt3"
  [Tt2] -> Bus Creator1/3  "Tt2"
  Bus Creator1/1 -> [InputVars_TestBench]
  [MN] -> Bus Creator1/2  "MN"
  [Altitude] -> Bus Creator1/1  "Altitude"
  Faults/1 -> [Faults]
  [Faults] -> S-Function1/4
  [Tt2] -> Scope8/1  "Nmech"
  [Pt3] -> Add2/1, Scope7/1  "Nmech"
  [Tt4] -> Scope6/1  "Nmech"
  Demux4/4 -> Scope8/2
  Demux4/3 -> Add2/2, Scope7/2
  Demux4/2 -> Scope6/2
  Demux4/1 -> Add1/2, Scope5/2
  [NMech] -> Add1/1, Scope5/1  "Nmech"
  [FuelLackModel] -> Demux4/1
  S-Function1/3 -> [FuelLackModel]
  [NormalModel] -> Demux3/1
  Add/1 -> Abs/1
  Abs/1 -> Scope9/1
  Add1/1 -> Abs1/1
  Abs1/1 -> Scope9/2
  Add2/1 -> Abs2/1
  Abs2/1 -> Product/1, Product/2
  Product/1 -> Scope10/1

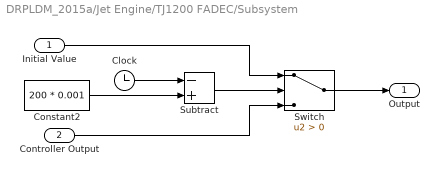
== system DRPLDM_2015a/Jet Engine/TJ1200 FADEC/Subsystem ==
  Initial Value : Inport
  Controller Output : Inport  Port=2
  Clock : Clock
  Constant2 : Constant  Value=200 * 0.001
  Subtract : Sum  Inputs=-+
  Switch : Switch  Criteria=u2 > Threshold
  Output : Outport
  wires:
  Subtract/1 -> Switch/2
  Initial Value/1 -> Switch/1
  Controller Output/1 -> Switch/3
  Switch/1 -> Output/1
  Clock/1 -> Subtract/1
  Constant2/1 -> Subtract/2

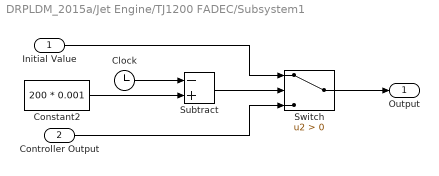
== system DRPLDM_2015a/Jet Engine/TJ1200 FADEC/Subsystem1 ==
  Initial Value : Inport
  Controller Output : Inport  Port=2
  Clock : Clock
  Constant2 : Constant  Value=200 * 0.001
  Subtract : Sum  Inputs=-+
  Switch : Switch  Criteria=u2 > Threshold
  Output : Outport
  wires:
  Constant2/1 -> Subtract/2
  Clock/1 -> Subtract/1
  Switch/1 -> Output/1
  Controller Output/1 -> Switch/3
  Initial Value/1 -> Switch/1
  Subtract/1 -> Switch/2

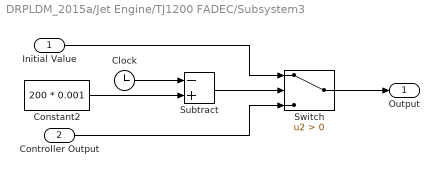
== system DRPLDM_2015a/Jet Engine/TJ1200 FADEC/Subsystem3 ==
  Initial Value : Inport
  Controller Output : Inport  Port=2
  Clock : Clock
  Constant2 : Constant  Value=200 * 0.001
  Subtract : Sum  Inputs=-+
  Switch : Switch  Criteria=u2 > Threshold
  Output : Outport
  wires:
  Constant2/1 -> Subtract/2
  Clock/1 -> Subtract/1
  Switch/1 -> Output/1
  Controller Output/1 -> Switch/3
  Initial Value/1 -> Switch/1
  Subtract/1 -> Switch/2

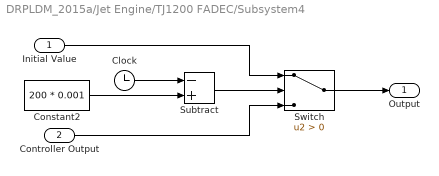
== system DRPLDM_2015a/Jet Engine/TJ1200 FADEC/Subsystem4 ==
  Initial Value : Inport
  Controller Output : Inport  Port=2
  Clock : Clock
  Constant2 : Constant  Value=200 * 0.001
  Subtract : Sum  Inputs=-+
  Switch : Switch  Criteria=u2 > Threshold
  Output : Outport
  wires:
  Subtract/1 -> Switch/2
  Initial Value/1 -> Switch/1
  Controller Output/1 -> Switch/3
  Switch/1 -> Output/1
  Clock/1 -> Subtract/1
  Constant2/1 -> Subtract/2

== matlab function DRPLDM_2015a/Jet Engine/MATLAB Function ==
  data: Time input; Bits output; StartTime input; StopTime input; IntRep output; SoftSim input
function [Bits,IntRep]  = fcn(Time, StartTime, StopTime, SoftSim)

    IntRep = 0;
    %Declares a static variable u
    persistent u;
        
    %Initiates the static variable u
    if isempty(u)
        u = zeros(1,length(StartTime)+ 1);
    end

    %Stores the bit indicating that thermocouples' fault simulation must be
    %performed by software
    u(end) = SoftSim;
    
    %Computes the SoftSim flat in int representation
    IntRep = u(end) * 2 ^ (length(u) - 1);
    
    %Executes loop verifying if Time is between StartTime and StopTime for
    %each individual fault setting. If true, fault must be simulated
    for i = 1:length(StartTime)
        
        if (Time < StopTime(i))&&(Time > StartTime(i))
            
            u(i) = 1;
            
        else
            
            u(i) = 0;
            
        end
        
        %Adds corresponding integer decimal term
        IntRep = IntRep + u(i) * 2^(i-1);
        
    end
    
Bits = u;
